simulink model "metoda_splotowa_2021b"  (R2021b)
settings: Solver=FixedStepAuto  StartTime=0.0  StopTime=20  FixedStep=step_size  RelTol=1e-3
undefined symbols (not defined in the file or in its folder): A, Ac, B, C, D, K, phi, phi_1, phi_2, phi_3, step_size, T_iD
libraries: SignalEditorBlockLib x1
settings Model: NumberOfSteps=10  Creator=janja  LastModifiedBy=janja
settings SolverCC: ConcurrentTasks=on  PositivePriorityOrder=on
settings OptimizationCC: BlockReduction=off  DefaultParameterBehavior=Inlined  OptimizeBlockIOStorage=off  EnhancedBackFolding=on  PassReuseOutputArgsThreshold=0  InitFltsAndDblsToZero=on  OptimizeBlockOrder=speed  DifferentSizesBufferReuse=on
settings DebuggingCC: TasksWithSamePriorityMsg=none  ParameterTunabilityLossMsg=error  UnderSpecifiedDimensionMsg=error
settings HardwareCC: TargetLongLongMode=on
settings SFSimCC: SimTargetLang=C++
settings RTWCC: BuildConfiguration=Faster Runs
settings CodeAppCC: OperatorAnnotations=on

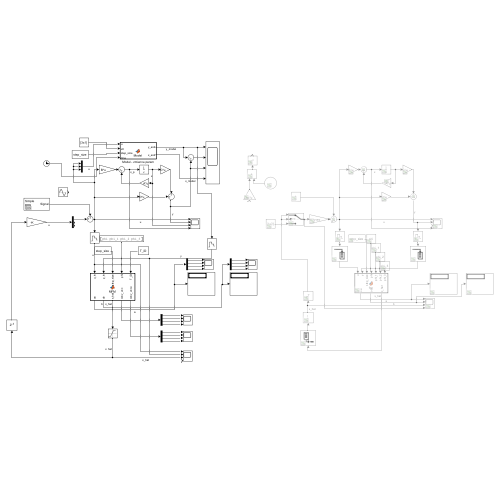
[thumbnail: Simulink's stored preview of the top-level diagram]
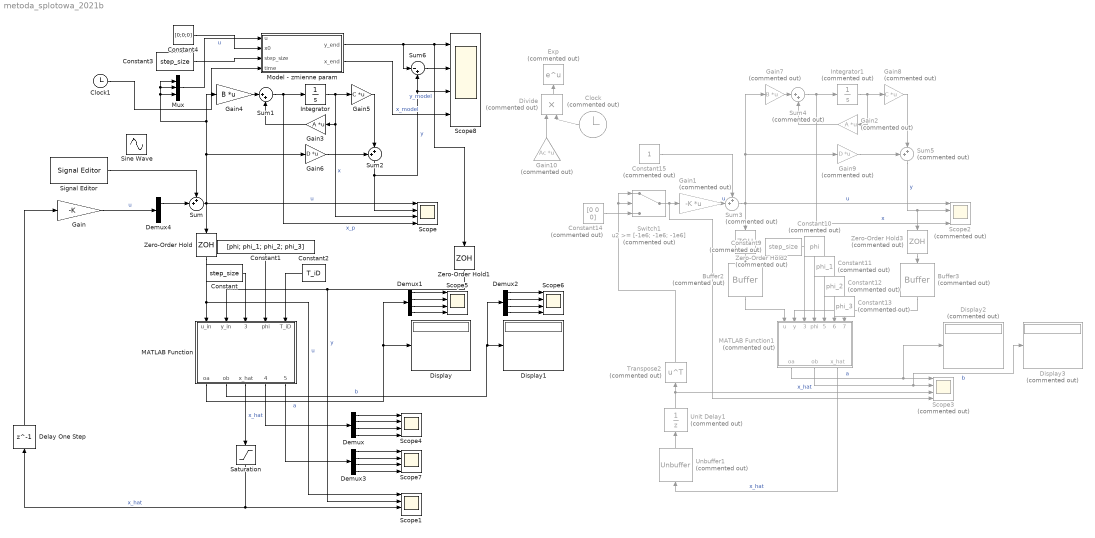
== system metoda_splotowa_2021b ==
  Buffer2 : Buffer  Commented=on  N=T_iD  V=T_iD-1  OutputFrames=off
  Buffer3 : Buffer  Commented=on  N=T_iD  V=T_iD-1  OutputFrames=off
  Clock : Clock  Commented=on
  Clock1 : Clock
  Constant : Constant  Value=step_size
  Constant1 : Constant  Value=[phi; phi_1; phi_2; phi_3]
  Constant10 : Constant  Commented=on  Value=phi
  Constant11 : Constant  Commented=on  Value=phi_1
  Constant12 : Constant  Commented=on  Value=phi_2
  Constant13 : Constant  Commented=on  Value=phi_3
  Constant14 : Constant  Commented=on  Value=[0 0 0]
  Constant15 : Constant  Commented=on
  Constant2 : Constant  Value=T_iD
  Constant3 : Constant  Value=step_size
  Constant4 : Constant  Value=[0;0;0]
  Constant9 : Constant  Commented=on  Value=step_size
  Delay One Step : Delay  DelayLength=1
  Demux{,1..3} (4 alike) : Demux
  Demux4 : Demux  Outputs=3
  Display : Display
  Display1 : Display
  Display2 : Display  Commented=on
  Display3 : Display  Commented=on
  Divide : Product  Commented=on  Inputs=**
  Exp : Math  Commented=on  SaturateOnIntegerOverflow=on
  Gain : Gain  Gain=-K
  Gain1 : Gain  Commented=on  Gain=-K  Multiplication=Matrix(K*u) (u vector)
  Gain10 : Gain  Commented=on  Gain=Ac  Multiplication=Matrix(K*u)
  Gain2 : Gain  Commented=on  Gain=A  Multiplication=Matrix(K*u)
  Gain3 : Gain  Gain=A  Multiplication=Matrix(K*u)
  Gain4 : Gain  Gain=B  Multiplication=Matrix(K*u)
  Gain5 : Gain  Gain=C  Multiplication=Matrix(K*u)
  Gain6 : Gain  Gain=D  Multiplication=Matrix(K*u)
  Gain7 : Gain  Commented=on  Gain=B  Multiplication=Matrix(K*u)
  Gain8 : Gain  Commented=on  Gain=C  Multiplication=Matrix(K*u)
  Gain9 : Gain  Commented=on  Gain=D  Multiplication=Matrix(K*u)
  Integrator : Integrator  InitialCondition=[0 0 0]
  Integrator1 : Integrator  Commented=on  InitialCondition=[0 0 0]
  MATLAB Function : MATLAB Function  TreatAsAtomicUnit=on
  MATLAB Function1 : MATLAB Function  Commented=on  TreatAsAtomicUnit=on
  Model - zmienne param : MATLAB Function  TreatAsAtomicUnit=on
  Mux : Mux  Inputs=3
  Saturation : Saturate  UpperLimit=4  LowerLimit=-4
  Scope{,1,4..8} (7 alike) : Scope  NumInputPorts=4
  Scope2 : Scope  Commented=on  NumInputPorts=4
  Scope3 : Scope  Commented=on  NumInputPorts=4
  Signal Editor : SignalEditorBlockLib/Signal Editor  FileName=custom_control.mat  ActiveScenario=Simple  ActiveSignal=Signal  IsBus=off  OutputBusObjectStr=Bus: BusObject  SampleTime=0  Interpolate=off  ZeroCross=off  OutputAfterFinalValue=Setting to zero  Unit=inherit  PreserveSignalName=on
  Sine Wave : Sin  SampleTime=0
  Sum : Sum  Inputs=++|
  Sum1 : Sum  Inputs=|++
  Sum2 : Sum  Inputs=++|
  Sum3 : Sum  Commented=on  Inputs=++|
  Sum4 : Sum  Commented=on  Inputs=|++
  Sum5 : Sum  Commented=on  Inputs=++|
  Sum6 : Sum  Inputs=|-+
  Switch1 : Switch  Commented=on  Threshold=[-1e6; -1e6; -1e6]
  Transpose2 : Math  Commented=on  Operator=transpose  OutputSignalType=real  SaturateOnIntegerOverflow=on
  Unbuffer1 : Unbuffer  Commented=on
  Unit Delay1 : UnitDelay  Commented=on  SampleTime=step_size  HasFrameUpgradeWarning=on
  Zero-Order Hold : ZeroOrderHold  SampleTime=step_size
  Zero-Order Hold1 : ZeroOrderHold  SampleTime=step_size
  Zero-Order Hold2 : ZeroOrderHold  Commented=on  SampleTime=step_size
  Zero-Order Hold3 : ZeroOrderHold  Commented=on  SampleTime=step_size
  wires:
  Integrator/1 -> Gain5/1, Scope/3, Gain3/1  "x"
  Gain4/1 -> Sum1/1
  Gain3/1 -> Sum1/2
  Sum1/1 -> Scope/4, Integrator/1  "x_p"
  Sum2/1 -> Sum6/2, Scope8/3, Scope/2  "y"
  Gain5/1 -> Sum2/2
  Gain6/1 -> Sum2/1
  Constant/1 -> MATLAB Function/3(step_size)
  MATLAB Function/2(ob) -> Demux2/1, Display1/1  "b"
  Constant1/1 -> MATLAB Function/4(phi)
  MATLAB Function/1(oa) -> Display/1, Demux1/1  "a"
  Sum/1 -> Scope/1, Zero-Order Hold/1, Gain6/1, Mux/3, Mux/2, Mux/1, Gain4/1  "u"
  Constant10/1 -> MATLAB Function1/4(phi)
  Buffer2/1 -> MATLAB Function1/1(u)
  Unit Delay1/1 -> Scope3/3, Transpose2/1  "x_hat"
  Constant11/1 -> MATLAB Function1/5(phi_1)
  Switch1/1 -> Scope3/4, Gain1/1
  Zero-Order Hold3/1 -> Buffer3/1
  Gain9/1 -> Sum5/1
  Zero-Order Hold2/1 -> Buffer2/1
  Buffer3/1 -> MATLAB Function1/2(y)
  MATLAB Function1/2(ob) -> Display3/1, Scope3/2  "b"
  Sum5/1 -> Zero-Order Hold3/1, Scope2/2  "y"
  Sum4/1 -> Scope2/4, Integrator1/1  "x"
  Gain2/1 -> Sum4/2
  Constant9/1 -> MATLAB Function1/3(step_size)
  Gain1/1 -> Sum3/2  "u"
  MATLAB Function1/1(oa) -> Display2/1, Scope3/1  "a"
  Constant12/1 -> MATLAB Function1/6(phi_2)
  Transpose2/1 -> Switch1/1, Switch1/2
  Unbuffer1/1 -> Unit Delay1/1
  MATLAB Function1/3(x_hat) -> Unbuffer1/1  "x_hat"
  Constant14/1 -> Switch1/3
  Gain8/1 -> Sum5/2
  Sum3/1 -> Gain9/1, Gain7/1, Scope2/1, Zero-Order Hold2/1  "u"
  Gain7/1 -> Sum4/1
  Constant13/1 -> MATLAB Function1/7(phi_3)
  Constant15/1 -> Sum3/1
  Integrator1/1 -> Gain8/1, Gain2/1
  MATLAB Function/3(x_hat) -> Saturation/1  "x_hat"
  Constant2/1 -> MATLAB Function/5(T_iD)
  MATLAB Function/4(conv_vec) -> Demux/1
  Demux/1 -> Scope4/1
  Demux/2 -> Scope4/2
  Demux/3 -> Scope4/3
  Demux/4 -> Scope4/4
  Demux2/1 -> Scope6/1
  Demux2/2 -> Scope6/2
  Demux2/3 -> Scope6/3
  Demux2/4 -> Scope6/4
  Zero-Order Hold/1 -> MATLAB Function/1(u_in), Scope1/1  "u"
  Zero-Order Hold1/1 -> Scope1/2, MATLAB Function/2(y_in)  "y"
  Demux1/1 -> Scope5/1
  Demux1/2 -> Scope5/2
  Demux1/3 -> Scope5/3
  Demux1/4 -> Scope5/4
  Demux3/1 -> Scope7/1
  Demux3/3 -> Scope7/3
  Demux3/2 -> Scope7/2
  Demux3/4 -> Scope7/4
  MATLAB Function/5(conv_vecu) -> Demux3/1
  Gain/1 -> Demux4/1  "u"
  Saturation/1 -> Scope1/3, Delay One Step/1  "x_hat"
  Demux4/1 -> Sum/2
  Delay One Step/1 -> Gain/1
  Divide/1 -> Exp/1
  Gain10/1 -> Divide/1
  Clock/1 -> Divide/2
  Signal Editor/1 -> Sum/1
  Constant3/1 -> Model - zmienne param/3(step_size)
  Constant4/1 -> Model - zmienne param/2(x0)
  Model - zmienne param/1(y_end) -> Sum6/1, Zero-Order Hold1/1, Scope8/1  "y_model"
  Mux/1 -> Model - zmienne param/1(u)  "u"
  Sum6/1 -> Scope8/2
  Model - zmienne param/2(x_end) -> Scope8/4  "x_model"
  Clock1/1 -> Model - zmienne param/4(time)

== matlab function metoda_splotowa_2021b/MATLAB Function1 ==
  data: u input; oa output; y input; step_size input; ob output; phi input; phi_1 input; phi_2 input; phi_3 input; x_hat output
function [oa, ob, x_hat]= fcn(u, y, step_size, phi, phi_1, phi_2, phi_3)

%splot y*phi u*phi
h=length(phi);
T_iD=length(u);
y0=zeros(T_iD-h+1,1);
y1=zeros(T_iD-h+1,1);
y2=zeros(T_iD-h+1,1);
y3=zeros(T_iD-h+1,1);
u0=zeros(T_iD-h+1,1);
u1=zeros(T_iD-h+1,1);
u2=zeros(T_iD-h+1,1);
u3=zeros(T_iD-h+1,1);
t_=0:step_size:((2*h-2)*step_size);
for t_h=h:T_iD
    y0(t_h-h+1)=trapz(t_,conv(y(t_h-h+1:t_h),phi),1);
    y1(t_h-h+1)=trapz(t_,conv(y(t_h-h+1:t_h),phi_1),1);
    y2(t_h-h+1)=trapz(t_,conv(y(t_h-h+1:t_h),phi_2),1);
    y3(t_h-h+1)=trapz(t_,conv(y(t_h-h+1:t_h),phi_3),1);
    u0(t_h-h+1)=trapz(t_,conv(u(t_h-h+1:t_h),phi),1);
    u1(t_h-h+1)=trapz(t_,conv(u(t_h-h+1:t_h),phi_1),1);
    u2(t_h-h+1)=trapz(t_,conv(u(t_h-h+1:t_h),phi_2),1);
    u3(t_h-h+1)=trapz(t_,conv(u(t_h-h+1:t_h),phi_3),1);
end
% size=length(u0);
t=((h-1)*step_size):step_size:((T_iD-1)*step_size);
%integ(y*u dt) h->T => y(T)u(T) - y(h)u(h) - integ(y'integ(u) dt) h->T
% y0_prim=diff(y0)/step_size;
% y1_prim=diff(y1)/step_size;
% y2_prim=diff(y2)/step_size;
% y3_prim=diff(y3)/step_size;
% u0_prim=diff(u0)/step_size;
% u1_prim=diff(u1)/step_size;
% u2_prim=diff(u2)/step_size;
% u3_prim=diff(u3)/step_size;
% y0_integ=trapz(t,y0(1:end-1),1);
% y1_integ=trapz(t,y1(1:end-1),1);
% y2_integ=trapz(t,y2(1:end-1),1);
% y3_integ=trapz(t,y3(1:end-1),1);
% u0_integ=trapz(t,u0(1:end-1),1);
% u1_integ=trapz(t,u1(1:end-1),1);
% u2_integ=trapz(t,u2(1:end-1),1);
% u3_integ=trapz(t,u3(1:end-1),1);

% g11=y0(end)*y0(end) -y0(1)*y0(1) -trapz(t,y0_prim.*y0_integ,1);
% g12=y0(end)*y1(end) -y0(1)*y1(1) -trapz(t,y0_prim.*y1_integ,1);
% g13=y0(end)*y2(end) -y0(1)*y2(1) -trapz(t,y0_prim.*y2_integ,1);
% g14=y0(end)*y3(end) -y0(1)*y3(1) -trapz(t,y0_prim.*y3_integ,1);
% g15=y0(end)*u0(end) -y0(1)*u0(1) -trapz(t,y0_prim.*u0_integ,1);
% g16=y0(end)*u1(end) -y0(1)*u1(1) -trapz(t,y0_prim.*u1_integ,1);
% g17=y0(end)*u2(end) -y0(1)*u2(1) -trapz(t,y0_prim.*u2_integ,1);
% g18=y0(end)*u3(end) -y0(1)*u3(1) -trapz(t,y0_prim.*u3_integ,1);
% 
% g21=y1(end)*y0(end) -y1(1)*y0(1) -trapz(t,y1_prim.*y0_integ,1);
% g22=y1(end)*y1(end) -y1(1)*y1(1) -trapz(t,y1_prim.*y1_integ,1);
% g23=y1(end)*y2(end) -y1(1)*y2(1) -trapz(t,y1_prim.*y2_integ,1);
% g24=y1(end)*y3(end) -y1(1)*y3(1) -trapz(t,y1_prim.*y3_integ,1);
% g25=y1(end)*u0(end) -y1(1)*u0(1) -trapz(t,y1_prim.*u0_integ,1);
% g26=y1(end)*u1(end) -y1(1)*u1(1) -trapz(t,y1_prim.*u1_integ,1);
% g27=y1(end)*u2(end) -y1(1)*u2(1) -trapz(t,y1_prim.*u2_integ,1);
% g28=y1(end)*u3(end) -y1(1)*u3(1) -trapz(t,y1_prim.*u3_integ,1);
% 
% g31=y2(end)*y0(end) -y2(1)*y0(1) -trapz(t,y2_prim.*y0_integ,1);
% g32=y2(end)*y1(end) -y2(1)*y1(1) -trapz(t,y2_prim.*y1_integ,1);
% g33=y2(end)*y2(end) -y2(1)*y2(1) -trapz(t,y2_prim.*y2_integ,1);
% g34=y2(end)*y3(end) -y2(1)*y3(1) -trapz(t,y2_prim.*y3_integ,1);
% g35=y2(end)*u0(end) -y2(1)*u0(1) -trapz(t,y2_prim.*u0_integ,1);
% g36=y2(end)*u1(end) -y2(1)*u1(1) -trapz(t,y2_prim.*u1_integ,1);
% g37=y2(end)*u2(end) -y2(1)*u2(1) -trapz(t,y2_prim.*u2_integ,1);
% g38=y2(end)*u3(end) -y2(1)*u3(1) -trapz(t,y2_prim.*u3_integ,1);
% 
% g41=y3(end)*y0(end) -y3(1)*y0(1) -trapz(t,y3_prim.*y0_integ,1);
% g42=y3(end)*y1(end) -y3(1)*y1(1) -trapz(t,y3_prim.*y1_integ,1);
% g43=y3(end)*y2(end) -y3(1)*y2(1) -trapz(t,y3_prim.*y2_integ,1);
% g44=y3(end)*y3(end) -y3(1)*y3(1) -trapz(t,y3_prim.*y3_integ,1);
% g45=y3(end)*u0(end) -y3(1)*u0(1) -trapz(t,y3_prim.*u0_integ,1);
% g46=y3(end)*u1(end) -y3(1)*u1(1) -trapz(t,y3_prim.*u1_integ,1);
% g47=y3(end)*u2(end) -y3(1)*u2(1) -trapz(t,y3_prim.*u2_integ,1);
% g48=y3(end)*u3(end) -y3(1)*u3(1) -trapz(t,y3_prim.*u3_integ,1);
% 
% g51=u0(end)*y0(end) -u0(1)*y0(1) -trapz(t,u0_prim.*y0_integ,1);
% g52=u0(end)*y1(end) -u0(1)*y1(1) -trapz(t,u0_prim.*y1_integ,1);
% g53=u0(end)*y2(end) -u0(1)*y2(1) -trapz(t,u0_prim.*y2_integ,1);
% g54=u0(end)*y3(end) -u0(1)*y3(1) -trapz(t,u0_prim.*y3_integ,1);
% g55=u0(end)*u0(end) -u0(1)*u0(1) -trapz(t,u0_prim.*u0_integ,1);
% g56=u0(end)*u1(end) -u0(1)*u1(1) -trapz(t,u0_prim.*u1_integ,1);
% g57=u0(end)*u2(end) -u0(1)*u2(1) -trapz(t,u0_prim.*u2_integ,1);
% g58=u0(end)*u3(end) -u0(1)*u3(1) -trapz(t,u0_prim.*u3_integ,1);
% 
% g61=u1(end)*y0(end) -u1(1)*y0(1) -trapz(t,u1_prim.*y0_integ,1);
% g62=u1(end)*y1(end) -u1(1)*y1(1) -trapz(t,u1_prim.*y1_integ,1);
% g63=u1(end)*y2(end) -u1(1)*y2(1) -trapz(t,u1_prim.*y2_integ,1);
% g64=u1(end)*y3(end) -u1(1)*y3(1) -trapz(t,u1_prim.*y3_integ,1);
% g65=u1(end)*u0(end) -u1(1)*u0(1) -trapz(t,u1_prim.*u0_integ,1);
% g66=u1(end)*u1(end) -u1(1)*u1(1) -trapz(t,u1_prim.*u1_integ,1);
% g67=u1(end)*u2(end) -u1(1)*u2(1) -trapz(t,u1_prim.*u2_integ,1);
% g68=u1(end)*u3(end) -u1(1)*u3(1) -trapz(t,u1_prim.*u3_integ,1);
% 
% g71=u2(end)*y0(end) -u2(1)*y0(1) -trapz(t,u2_prim.*y0_integ,1);
% g72=u2(end)*y1(end) -u2(1)*y1(1) -trapz(t,u2_prim.*y1_integ,1);
% g73=u2(end)*y2(end) -u2(1)*y2(1) -trapz(t,u2_prim.*y2_integ,1);
% g74=u2(end)*y3(end) -u2(1)*y3(1) -trapz(t,u2_prim.*y3_integ,1);
% g75=u2(end)*u0(end) -u2(1)*u0(1) -trapz(t,u2_prim.*u0_integ,1);
% g76=u2(end)*u1(end) -u2(1)*u1(1) -trapz(t,u2_prim.*u1_integ,1);
% g77=u2(end)*u2(end) -u2(1)*u2(1) -trapz(t,u2_prim.*u2_integ,1);
% g78=u2(end)*u3(end) -u2(1)*u3(1) -trapz(t,u2_prim.*u3_integ,1);
% 
% g81=u3(end)*y0(end) -u3(1)*y0(1) -trapz(t,u3_prim.*y0_integ,1);
% g82=u3(end)*y1(end) -u3(1)*y1(1) -trapz(t,u3_prim.*y1_integ,1);
% g83=u3(end)*y2(end) -u3(1)*y2(1) -trapz(t,u3_prim.*y2_integ,1);
% g84=u3(end)*y3(end) -u3(1)*y3(1) -trapz(t,u3_prim.*y3_integ,1);
% g85=u3(end)*u0(end) -u3(1)*u0(1) -trapz(t,u3_prim.*u0_integ,1);
% g86=u3(end)*u1(end) -u3(1)*u1(1) -trapz(t,u3_prim.*u1_integ,1);
% g87=u3(end)*u2(end) -u3(1)*u2(1) -trapz(t,u3_prim.*u2_integ,1);
% g88=u3(end)*u3(end) -u3(1)*u3(1) -trapz(t,u3_prim.*u3_integ,1);

g11=trapz(t,y0.*y0,1);
g12=trapz(t,y0.*y1,1);
g13=trapz(t,y0.*y2,1);
g14=trapz(t,y0.*y3,1);
g15=trapz(t,y0.*u0,1);
g16=trapz(t,y0.*u1,1);
g17=trapz(t,y0.*u2,1);
g18=trapz(t,y0.*u3,1);

g21=trapz(t,y1.*y0,1);
g22=trapz(t,y1.*y1,1);
g23=trapz(t,y1.*y2,1);
g24=trapz(t,y1.*y3,1);
g25=trapz(t,y1.*u0,1);
g26=trapz(t,y1.*u1,1);
g27=trapz(t,y1.*u2,1);
g28=trapz(t,y1.*u3,1);

g31=trapz(t,y2.*y0,1);
g32=trapz(t,y2.*y1,1);
g33=trapz(t,y2.*y2,1);
g34=trapz(t,y2.*y3,1);
g35=trapz(t,y2.*u0,1);
g36=trapz(t,y2.*u1,1);
g37=trapz(t,y2.*u2,1);
g38=trapz(t,y2.*u3,1);

g41=trapz(t,y3.*y0,1);
g42=trapz(t,y3.*y1,1);
g43=trapz(t,y3.*y2,1);
g44=trapz(t,y3.*y3,1);
g45=trapz(t,y3.*u0,1);
g46=trapz(t,y3.*u1,1);
g47=trapz(t,y3.*u2,1);
g48=trapz(t,y3.*u3,1);

g51=trapz(t,u0.*y0,1);
g52=trapz(t,u0.*y1,1);
g53=trapz(t,u0.*y2,1);
g54=trapz(t,u0.*y3,1);
g55=trapz(t,u0.*u0,1);
g56=trapz(t,u0.*u1,1);
g57=trapz(t,u0.*u2,1);
g58=trapz(t,u0.*u3,1);

% g61=trapz(t,u1.*y0,1);
% g62=trapz(t,u1.*y1,1);
% g63=trapz(t,u1.*y2,1);
% g64=trapz(t,u1.*y3,1);
% g65=trapz(t,u1.*u0,1);
% g66=trapz(t,u1.*u1,1);
% g67=trapz(t,u1.*u2,1);
% g68=trapz(t,u1.*u3,1);
% 
% g71=trapz(t,u2.*y0,1);
% g72=trapz(t,u2.*y1,1);
% g73=trapz(t,u2.*y2,1);
% g74=trapz(t,u2.*y3,1);
% g75=trapz(t,u2.*u0,1);
% g76=trapz(t,u2.*u1,1);
% g77=trapz(t,u2.*u2,1);
% g78=trapz(t,u2.*u3,1);
% 
% g81=trapz(t,u3.*y0,1);
% g82=trapz(t,u3.*y1,1);
% g83=trapz(t,u3.*y2,1);
% g84=trapz(t,u3.*y3,1);
% g85=trapz(t,u3.*u0,1);
% g86=trapz(t,u3.*u1,1);
% g87=trapz(t,u3.*u2,1);
% g88=trapz(t,u3.*u3,1);

% G=[g11 g12 g13 g14 -g15 -g16 -g17 -g18;
%    g21 g22 g23 g24 -g25 -g26 -g27 -g28;
%    g31 g32 g33 g34 -g35 -g36 -g37 -g38;
%    g41 g42 g43 g44 -g45 -g46 -g47 -g48;
%    g51 g52 g53 g54 -g55 -g56 -g57 -g58;
%    g61 g62 g63 g64 -g65 -g66 -g67 -g68;
%    g71 g72 g73 g74 -g75 -g76 -g77 -g78;
%    g81 g82 g83 g84 -g85 -g86 -g87 -g88];

G=[g11 g12 g13 g14 -g15 ;
   g21 g22 g23 g24 -g25 ;
   g31 g32 g33 g34 -g35 ;
   g41 g42 g43 g44 -g45 ;
   g51 g52 g53 g54 -g55 ];

[V, D]=eig(G);
I=[0 0 0 0 0];
M=[1e6 1e6 1e6 1e6 1e6];
D=real(D);
V=real(V);
for j=1:length(D)
        for i=1:length(D)
            if i==j
                M(j)=D(i,j);
                I(j)=i;
            end
        end
end
ind=1;
for i=1:length(M)
    if abs(M(i))>1e-10 && min(M)==M(i)
        ind=i;
    end
end
%mogę identyfikować wszystkie a i b, później najwyżej się wyzerują
% oa=[V(4,1) V(3,1) V(2,1) V(1,1)];
% ob=[V(8,1) V(7,1) V(6,1) V(5,1)];

oa=[V(4,ind) V(3,ind) V(2,ind) V(1,ind)];
ob=[V(5,ind)];

H1=1/oa(1)*[oa(3) oa(2) oa(1) 0;
            oa(2) oa(1) 0 0;
            oa(1) 0 0 0];
% H2=1/oa(1)*[ob(3) ob(2) 0;
%             ob(2) 0 0;
%             0 0 0];
H2=1/oa(1)*[ob(1) 0 0;
            0 0 0;
            0 0 0];

% x_hat=real(transpose(H1*[y0';y1';y2';y3']-H2*[u0';u1';u2']));
x_hat=real(transpose(H1*[y0';y1';y2';y3']-H2*[u0';u1';u2']));

== matlab function metoda_splotowa_2021b/MATLAB Function ==
  data: u_in input; y_in input; step_size input; phi input; T_iD input; oa output size=4; ob output size=4; x_hat output size=3; conv_vec output size=[4 1]; conv_vecu output size=[4 1]
function [oa, ob, x_hat, conv_vec, conv_vecu] = MFM(u_in, y_in, step_size, phi, T_iD)
persistent u_buff_local y_buff_local y0 y1 y2 y3 u0 u1 u2 u3 a0_buff a1_buff a2_buff a3_buff b0_buff
    oa=[0 0 0 0]';
    ob=[0 0 0 0]';
    x_hat=[0 0 0]';
    phi_0=phi(1,:)';
    phi_1=phi(2,:)';
    phi_2=phi(3,:)';
    phi_3=phi(4,:)';
    conv_vec=[0 0 0 0]';
    conv_vecu=[0 0 0 0]';

%splot y*phi u*phi
h=length(phi_0);
if isempty(u_buff_local)
   u_buff_local=0;
   y_buff_local=0;
    y0=0;
    y1=0;
    y2=0;
    y3=0;
    u0=0;
    u1=0;
    u2=0;
    u3=0;
    a0_buff=0;
    a1_buff=0;
    a2_buff=0;
    a3_buff=0;
    b0_buff=0;
else
    u_buff_local=[u_buff_local; u_in];
    y_buff_local=[y_buff_local; y_in];
    y0 = [y0; 0];
    y1 = [y1; 0];
    y2 = [y2; 0];
    y3 = [y3; 0];
    u0 = [u0; 0];
    u1 = [u1; 0];
    u2 = [u2; 0];
    u3 = [u3; 0];
    len_u=length(u_buff_local);
    len_y=length(y_buff_local);
    if len_u>=h && len_y>=h
        if len_u>T_iD && len_y>T_iD
            u_buff_local=u_buff_local(end-T_iD+1:end);
            y_buff_local=y_buff_local(end-T_iD+1:end);
        end
        if len_u>T_iD-h && len_y>T_iD-h
            y0 = y0(end-T_iD+h+1:end);
            y1 = y1(end-T_iD+h+1:end);
            y2 = y2(end-T_iD+h+1:end);
            y3 = y3(end-T_iD+h+1:end);
            u0 = u0(end-T_iD+h+1:end);
            u1 = u1(end-T_iD+h+1:end);
            u2 = u2(end-T_iD+h+1:end);
            u3 = u3(end-T_iD+h+1:end);
                        
        end
        u=u_buff_local;
        y=y_buff_local;
%         y0=zeros(length(y_buff_local)-h+1,1);
%         y1=zeros(length(y_buff_local)-h+1,1);
%         y2=zeros(length(y_buff_local)-h+1,1);
%         y3=zeros(length(y_buff_local)-h+1,1);
%         u0=zeros(length(u_buff_local)-h+1,1);
%         u1=zeros(length(u_buff_local)-h+1,1);
%         u2=zeros(length(u_buff_local)-h+1,1);
%         u3=zeros(length(u_buff_local)-h+1,1);
        t_=0:step_size:((h-1)*step_size);
%         for t_h=h:length(y)
%             y0(t_h-h+1)=trapz(t_,(y(t_h-h+1:t_h).*flipud(phi_0)),1);
%             y1(t_h-h+1)=trapz(t_,(y(t_h-h+1:t_h).*flipud(phi_1)),1);
%             y2(t_h-h+1)=trapz(t_,(y(t_h-h+1:t_h).*flipud(phi_2)),1);
%             y3(t_h-h+1)=trapz(t_,(y(t_h-h+1:t_h).*flipud(phi_3)),1);
%             u0(t_h-h+1)=trapz(t_,(u(t_h-h+1:t_h).*flipud(phi_0)),1);
%             u1(t_h-h+1)=trapz(t_,(u(t_h-h+1:t_h).*flipud(phi_1)),1);
%             u2(t_h-h+1)=trapz(t_,(u(t_h-h+1:t_h).*flipud(phi_2)),1);
%             u3(t_h-h+1)=trapz(t_,(u(t_h-h+1:t_h).*flipud(phi_3)),1);
%         end

%%persistent variables
        y0(end)=trapz(t_,(y(end-h+1:end).*flipud(phi_0)),1);
        y1(end)=trapz(t_,(y(end-h+1:end).*flipud(phi_1)),1);
        y2(end)=trapz(t_,(y(end-h+1:end).*flipud(phi_2)),1);
        y3(end)=trapz(t_,(y(end-h+1:end).*flipud(phi_3)),1);
        u0(end)=trapz(t_,(u(end-h+1:end).*flipud(phi_0)),1);
        u1(end)=trapz(t_,(u(end-h+1:end).*flipud(phi_1)),1);
        u2(end)=trapz(t_,(u(end-h+1:end).*flipud(phi_2)),1);
        u3(end)=trapz(t_,(u(end-h+1:end).*flipud(phi_3)),1);

        % y0=fliplr(y0);
        % y1=fliplr(y1);
        % y2=fliplr(y2);
        % y3=fliplr(y3);
        % 
        % u0=fliplr(u0);
        % u1=fliplr(u1);
        % u2=fliplr(u2);
        % u3=fliplr(u3);

%         for t_h=h:length(y)
%             y0(t_h-h+1)=trapz(t_,conv(y(t_h-h+1:t_h),phi_0),1);
%             y1(t_h-h+1)=trapz(t_,conv(y(t_h-h+1:t_h),phi_1),1);
%             y2(t_h-h+1)=trapz(t_,conv(y(t_h-h+1:t_h),phi_2),1);
%             y3(t_h-h+1)=trapz(t_,conv(y(t_h-h+1:t_h),phi_3),1);
%             u0(t_h-h+1)=trapz(t_,conv(u(t_h-h+1:t_h),phi_0),1);
%             u1(t_h-h+1)=trapz(t_,conv(u(t_h-h+1:t_h),phi_1),1);
%             u2(t_h-h+1)=trapz(t_,conv(u(t_h-h+1:t_h),phi_2),1);
%             u3(t_h-h+1)=trapz(t_,conv(u(t_h-h+1:t_h),phi_3),1);
%         end

%         y0=conv(y(end-h+1:end),phi_0);
%         y1=conv(y(end-h+1:end),phi_1);
%         y2=conv(y(end-h+1:end),phi_2);
%         y3=conv(y(end-h+1:end),phi_3);
%         u0=conv(u(end-h+1:end),phi_0);
%         u1=conv(u(end-h+1:end),phi_1);
%         u2=conv(u(end-h+1:end),phi_2);
%         u3=conv(u(end-h+1:end),phi_3);
        conv_vec=[y0(end) y1(end) y2(end) y3(end)]';
        conv_vecu=[u0(end) u1(end) u2(end) u3(end)]';
        % size=length(u0);
        t=0:step_size:((length(y0)-1)*step_size);
        %integ(y*u dt) h->T => y(T)u(T) - y(h)u(h) - integ(y'integ(u) dt) h->T
        
        g11=dot(y0,y0);
        g12=dot(y0,y1);
        g13=dot(y0,y2);
        g14=dot(y0,y3);
        g15=dot(y0,u0);
        g16=dot(y0,u1);
        g17=dot(y0,u2);
        g18=dot(y0,u3);
        
%         g21=dot(y1,y0);
        g22=dot(y1,y1);
        g23=dot(y1,y2);
        g24=dot(y1,y3);
        g25=dot(y1,u0);
        g26=dot(y1,u1);
        g27=dot(y1,u2);
        g28=dot(y1,u3);
        
%         g31=dot(y2,y0,1);
%         g32=dot(y2,y1,1);
        g33=dot(y2,y2);
        g34=dot(y2,y3);
        g35=dot(y2,u0);
        g36=dot(y2,u1);
        g37=dot(y2,u2);
        g38=dot(y2,u3);
        
%         g41=dot(y3,y0,1);
%         g42=dot(y3,y1,1);
%         g43=dot(y3,y2,1);
        g44=dot(y3,y3);
        g45=dot(y3,u0);
        g46=dot(y3,u1);
        g47=dot(y3,u2);
        g48=dot(y3,u3);
        
%         g51=dot(u0,y0,1);
%         g52=dot(u0,y1,1);
%         g53=dot(u0,y2,1);
%         g54=dot(u0,y3,1);
        g55=dot(u0,u0);
        g56=dot(u0,u1);
        g57=dot(u0,u2);
        g58=dot(u0,u3);
        
        % g61=dot(u1,y0,1);
        % g62=dot(u1,y1,1);
        % g63=dot(u1,y2,1);
        % g64=dot(u1,y3,1);
        % g65=dot(u1,u0,1);
        g66=dot(u1,u1);
        g67=dot(u1,u2);
        g68=dot(u1,u3);
        % 
        % g71=dot(u2,y0,1);
        % g72=dot(u2,y1,1);
        % g73=dot(u2,y2,1);
        % g74=dot(u2,y3,1);
        % g75=dot(u2,u0,1);
        % g76=dot(u2,u1,1);
        g77=dot(u2,u2);
        g78=dot(u2,u3);
        % 
        % g81=dot(u3,y0,1);
        % g82=dot(u3,y1,1);
        % g83=dot(u3,y2,1);
        % g84=dot(u3,y3,1);
        % g85=dot(u3,u0,1);
        % g86=dot(u3,u1,1);
        % g87=dot(u3,u2,1);
        g88=dot(u3,u3);
        
        G=[g11 g12 g13 g14 -g15 -g16 -g17 -g18;
           g12 g22 g23 g24 -g25 -g26 -g27 -g28;
           g13 g23 g33 g34 -g35 -g36 -g37 -g38;
           g14 g24 g34 g44 -g45 -g46 -g47 -g48;
           -g15 -g25 -g35 -g45 g55 g56 g57 g58;
           -g16 -g26 -g36 -g46 g56 g66 g67 g68;
           -g17 -g27 -g37 -g47 g57 g67 g77 g78;
           -g18 -g28 -g38 -g48 g58 g68 g78 g88];
        
%         G=[g11 g12 g13 g14 -g15 ;
%            g12 g22 g23 g24 -g25 ;
%            g13 g23 g33 g34 -g35 ;
%            g14 g24 g34 g44 -g45 ;
%            -g15 -g25 -g35 -g45 g55 ];
        
        [V, D]=eig(G);
        V=abs(V);
        I=[0 0 0 0 0 0 0 0];
        M=[1e6 1e6 1e6 1e6 1e6 1e6 1e6 1e6];
        D=real(D);
        V=real(V);
        for j=1:length(D)
            for i=1:length(D)
                if i==j
                    M(j)=D(i,j);
                    I(j)=i;
                end
            end
        end
        ind=1;
        temp_min=1e6;
        for i=1:length(M)
            if  M(i)<temp_min %&& abs(M(i))>1e-10 
                ind=i;
                temp_min=M(ind);
            end
        end
        %mogę identyfikować wszystkie a i b, później najwyżej się wyzerują
        oa=[V(4,ind) V(3,ind) V(2,ind) V(1,ind)]';
        ob=[V(8,ind) V(7,ind) V(6,ind) V(5,ind)]';
%         V=abs(V);
% if length(y_buff_local)>5000
%         a0_buff(end)=V(1,ind);
%         a1_buff(end)=V(2,ind);
%         a2_buff(end)=V(3,ind);
%         a3_buff(end)=V(4,ind);
%         b0_buff(end)=V(5,ind);
% 
%         mean_window=h/2;
%         if length(a0_buff)>mean_window
%             a0_buff=a0_buff(end-mean_window+1:end);
%             a1_buff=a1_buff(end-mean_window+1:end);
%             a2_buff=a2_buff(end-mean_window+1:end);
%             a3_buff=a3_buff(end-mean_window+1:end);
%             b0_buff=b0_buff(end-mean_window+1:end);
%         end
% 
%         % oa(4)=mean(a0_buff);
%         % oa(3)=mean(a1_buff);
%         % oa(2)=mean(a2_buff);
%         % oa(1)=mean(a3_buff);
%         % ob(4)=mean(b0_buff);
% 
%         a0_buff(end+1)=0;
%         a1_buff(end+1)=0;
%         a2_buff(end+1)=0;
%         a3_buff(end+1)=0;
%         b0_buff(end+1)=0;
% end

        H1=1/oa(1)*[oa(3) oa(2) oa(1) 0;
                    oa(2) oa(1) 0 0;
                    oa(1) 0 0 0;];
        H2=1/oa(4)*[ob(3) ob(2) 0;
                    ob(2) 0 0;
                    0 0 0];
        % H2=1/oa(1)*[ob(3) 0 0;
        %             0 0 0;
        %             0 0 0];
        
        x_temp=real(H1*[y0(end);y1(end);y2(end);y3(end)]-H2*[u0(end);u1(end);u2(end)]);
        x_hat=x_temp;
    end
end

== matlab function metoda_splotowa_2021b/Model - zmienne param ==
  settings: updateMethod=DISCRETE
  data: u input size=[3 1]; y_end output; x0 input; step_size input; x_end output; time input
function [y_end,x_end] = Model(u,x0,step_size,time)

persistent x x_p L M

if isempty(x)
    x = x0;                % Set initial state
    x_p = x0;
    L=1;
    M=[1 6 2 1];
    % y=[0 0 0];
end

if time>10
    % L=L+0.001;
    M(2)=5;
    M(3)=3;
    % M(4)=M(4)+0.001;
end

[A,B,C,D]=tf2ss(L,M);

% Perform the system simulation:

% for n=1:Ns           % Iterate through time
  y = C*x_p + D*u; % Output for time n-1
  x(:,end) = A*x_p + B*u';    % State transitions to time n
  x = [x [0;0;0]];
  x_p = trapz(step_size,x(:,1:end-1),2);
% end
y_end=y(3);
x_end=x_p;
